simulink model "Lab3"  (R2022b)
settings: Solver=VariableStepAuto  StartTime=0.0  StopTime=50  MaxStep=0.02  RelTol=1e-3  AbsTol=1e-6
settings Model: Creator=vise  LastModifiedBy=David Mendoza
settings SolverCC: AutoScaleAbsTol=off  AlgebraicLoopSolver=TrustRegion
settings DataIOCC: SaveFormat=Array  SignalLoggingSaveFormat=ModelDataLogs  ReturnWorkspaceOutputs=off
settings OptimizationCC: BlockReduction=off  BooleanDataType=off  ExpressionDepthLimit=2147483647  InitFltsAndDblsToZero=on  LifeSpan=inf
settings DebuggingCC: SaveWithParameterizedLinksMsg=none  UnderspecifiedInitializationDetection=Classic  MergeDetectMultiDrivingBlocksExec=none  SignalResolutionControl=TryResolveAllWithWarning  MultiTaskDSMMsg=warning  MultiTaskCondExecSysMsg=none  FcnCallInpInsideContextMsg=warning  UnconnectedInputMsg=warning  UnconnectedOutputMsg=warning  UnconnectedLineMsg=warning  StateNameClashWarn=warning  SFUnexpectedBacktrackingDiag=warning  SFNoUnconditionalDefaultTransitionDiag=warning  SFExecutionAtInitializationDiag=none  SFMachineParentedDataDiag=warning  ArithmeticOperatorsInVariantConditions=warning
settings HardwareCC: ProdBitPerPointer=32  ProdBitPerSizeT=32  ProdBitPerPtrDiffT=32  ProdLargestAtomicFloat=None  ProdIntDivRoundTo=Undefined  ProdEndianess=Unspecified  ProdWordSize=32  ProdHWDeviceType=32-bit Generic  TargetUnknown=on
settings ModelReferenceCC: EnableRefExpFcnMdlSchedulingChecks=on  PropagateSignalLabelsOutOfModel=off
settings SFSimCC: SimUseLocalCustomCode=off  CustomCodeUndefinedFunction=UseInterfaceOnly
settings RTWCC: TemplateMakefile=grt_unix.tmf  RTWUseLocalCustomCode=off
settings CodeAppCC: StateflowObjectComments=on
settings GRTTargetCC: TargetLangStandard=C89/C90 (ANSI)  CombineOutputUpdateFcns=off  GRTInterface=on
settings ConfigComp: CovMetricSettings=dw  CovSaveCumulativeToWorkspaceVar=on  CovSaveSingleToWorkspaceVar=on  CovExternalEMLEnable=off

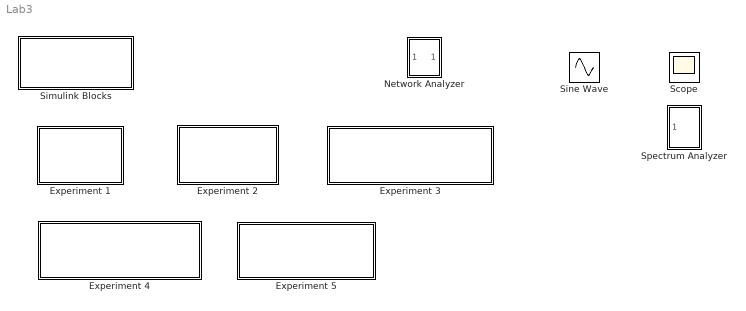
== system Lab3 ==
  Experiment 1 : Subsystem  mask(Waveform Synthesizer){}
      settings: OpenFcn=lab3Synth
      mask Display: disp('Synthesizer')
  Experiment 2 : Subsystem  mask(Modulator){}
      settings: OpenFcn=lab3Mod
      mask Display: disp('Modulator')
  Experiment 3 : Subsystem  mask(CT System Analysis/Network Analyzer){}
      settings: OpenFcn=lab3CTSys1
      mask Display: disp('CT System Analysis using\n a Network Analyzer')
  Experiment 4 : Subsystem  mask(CT System Analysis/Unit Step){}
      settings: OpenFcn=lab3CTSys2
      mask Display: disp('CT System Analysis using\n a Unit Step')
  Experiment 5 : Subsystem  mask(DT System Analysis){}
      settings: OpenFcn=lab3DTSys
      mask Display: disp('DT System Analysis')
  Network Analyzer : Subsystem  mask(Network Analyzer){MaskParam1=256, MaskParam2=0.1}
      mask prompts: MaskParam1 "Number of sample points:"; MaskParam2 "Sampling period (sec):"
      mask init:
      | max_freq=0.9*pi/MaskParam2;N=MaskParam1;T_s=MaskParam2;const=2*pi/(MaskParam1*MaskParam2);window1=0.5*MaskParam1*MaskParam2;window2=MaskParam1*MaskParam2;
      mask Help: Estimates frequency response of system using chirp input. Used for EE438. See Prof. Bouman.
      mask Display: plot(0,0,100,100,[11,93,93,11,11],[90,90,40,40,90],[80,60,40,20],[50,79,50,80])
  Scope : Scope
  Simulink Blocks : Subsystem  mask(Waveform Synthesizer){}
      settings: OpenFcn=simulink
      mask Display: disp('Full Block Library')
  Sine Wave : Sin  Frequency=7*pi  SampleTime=0
  Spectrum Analyzer : Subsystem  mask(Spectrum analyzer.){N=2048, T_s=0.02, plot_period=10}
      mask prompts: N "Number of sample points:"; T_s "Sampling period (sec):"; plot_period "Plotting Period (sec):"
      mask Help: EE438 Lab utility; See Prof. Bouman.
      mask Display: plot(0,0,100,100,[14,91,91,14,14],[86,86,40,40,86],[85,82,80,79,75,67,63,60,57,53,41,36,33,27,24],[49,50,53,50,49,51,54,66,54,50,50,52,81,51,49])

== system Lab3/Experiment 1 ==

== system Lab3/Experiment 2 ==

== system Lab3/Experiment 3 ==

== system Lab3/Experiment 4 ==

== system Lab3/Experiment 5 ==

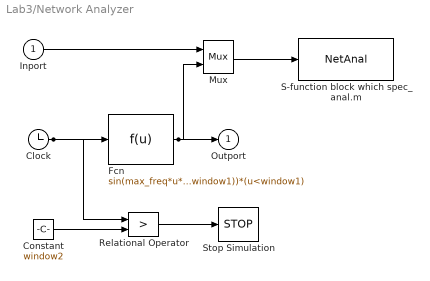
== system Lab3/Network Analyzer ==
  Inport : Inport
  Clock : Clock
  Constant : Constant  Value=window2
  Fcn : Fcn  Expr=sin(max_freq*u*u/(2*window1))*(0.54+0.46*cos(pi*u/window1))*(u<window1)
  Mux : Mux  Inputs=2
  Relational Operator : RelationalOperator  Operator=>
  S-function block which spec_anal.m : S-Function  FunctionName=NetAnal  Parameters=N,T_s  SFunctionDeploymentMode=off  EnableBusSupport=off
  Stop Simulation : Stop
  Outport : Outport  InitialOutput=0
  wires:
  Inport/1 -> Mux/1
  Fcn/1 -> Mux/2, Outport/1
  Mux/1 -> S-function block which spec_anal.m/1
  Clock/1 -> Fcn/1, Relational Operator/1
  Constant/1 -> Relational Operator/2
  Relational Operator/1 -> Stop Simulation/1

== system Lab3/Simulink Blocks ==

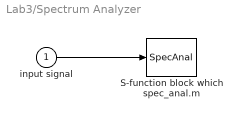
== system Lab3/Spectrum Analyzer ==
  input signal : Inport
  S-function block which spec_anal.m : S-Function  FunctionName=SpecAnal  Parameters=N,T_s,plot_period  SFunctionDeploymentMode=off  EnableBusSupport=off
  wires:
  input signal/1 -> S-function block which spec_anal.m/1
